simulink model "microgridbelbic"  (R2019a)
settings: Solver=VariableStepAuto  StartTime=0.0  StopTime=6  RelTol=1e-3
undefined symbols (not defined in the file): DiscIntNeverNeededParam, fdesignblkfcn, gcbh, Hydride, Metal, Nickel
libraries: powerlib x242, powerlib_extras x28, BELBICtoolbox x4, dsparch4 x1, electricdrivelib x1, simulink x1, sps_avr x1, powerlib_meascontrol x1, re_lib x1
(part 1 of 4)
settings Model: Creator=pavan  LastModifiedBy=pavan

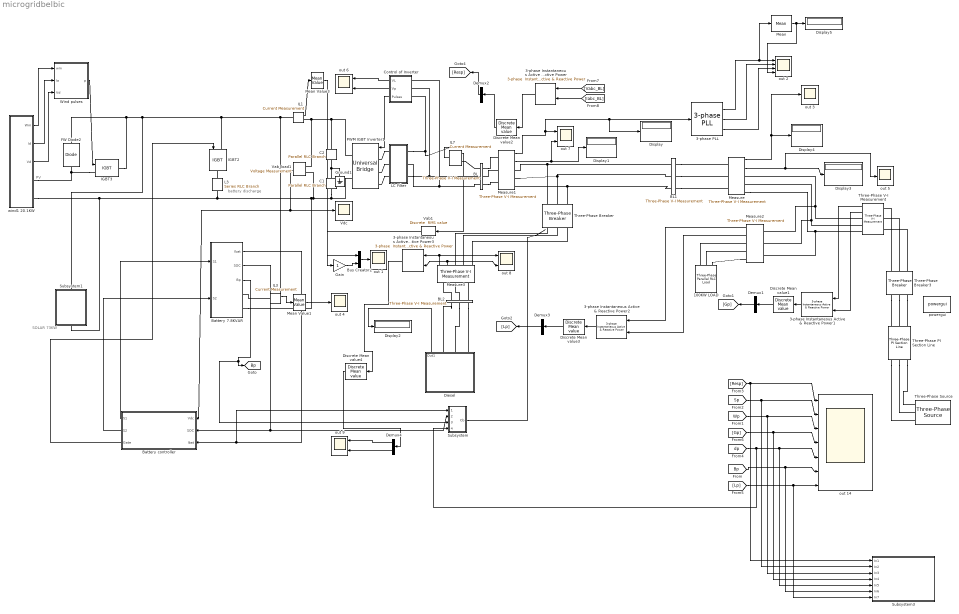
== system microgridbelbic ==
  note: SOLAR 73KW
  note: PV
  note: battery discharge
  100KW LOAD : powerlib/Elements/Three-Phase Parallel RLC Load  LConnTagsString=A|B|C  Configuration=Y (grounded)  NominalVoltage=400  Vabc=[1e3 1e3 1e3]  Vabcp=[1e3 1e3 1e3]  NominalFrequency=50  UnbalancedPower=off  ActivePower=80000  InductivePower=0  CapacitivePower=0  Pabc=[10e3 9e3 11e3]  QLabc=[100 90 110]  QCabc=[100 90 110]  Pabcp=[10e3 9e3 11e3]  QLabcp=[100 90 110]  QCabcp=[100 90 110]  Measurements=None  LoadType=constant Z
      settings: SourceProductName=Simscape Electrical
  3-phase Instantaneous Active & Reactive Power{,1..3} (4 alike) : powerlib_extras/Measurements/3-phase  Instantaneous  Active & Reactive Power
      settings: SourceProductName=Simscape Electrical  SourceProductBaseCode=PS
  3-phase PLL : powerlib_extras/Control  Blocks/3-phase PLL  Par_Init=[0 50]  ParK=[ 180 3200 1 ]  AGC=off
      settings: SourceProductName=Simscape Electrical  SourceProductBaseCode=PS
  BL : powerlib/Measurements/Three-Phase V-I Measurement  VoltageMeasurement=phase-to-ground  SetLabelV=on  LabelV=Vabc_BL1  Vpu=off  VpuLL=off  CurrentMeasurement=yes  SetLabelI=on  LabelI=Iabc_BL1  Ipu=off  Pbase=100e6  Vbase=500e3  OutputType=Magnitude  PhasorSimulation=off  PSBequivalent=0
      settings: SourceProductName=Simscape Electrical
  BL1 : powerlib/Measurements/Three-Phase V-I Measurement  VoltageMeasurement=phase-to-ground  SetLabelV=on  LabelV=Vabc_BL  Vpu=off  VpuLL=off  CurrentMeasurement=yes  SetLabelI=on  LabelI=Iabc_BL  Ipu=off  Pbase=100e6  Vbase=500e3  OutputType=Magnitude  PhasorSimulation=off  PSBequivalent=0
      settings: SourceProductName=Simscape Electrical
  BL2 : powerlib/Measurements/Three-Phase V-I Measurement  VoltageMeasurement=phase-to-ground  SetLabelV=on  LabelV=Vabc_BL2  Vpu=off  VpuLL=off  CurrentMeasurement=yes  SetLabelI=on  LabelI=Iabc_BL2  Ipu=off  Pbase=100e6  Vbase=500e3  OutputType=Magnitude  PhasorSimulation=off  PSBequivalent=0
      settings: SourceProductName=Simscape Electrical
  Battery controller : Subsystem
  "Battery 7.8KVAR " : Subsystem
  Bus Creator2 : BusCreator  Inputs=2
  C1 : powerlib/Elements/Parallel RLC Branch  LConnTagsString=a  RConnTagsString=__new0  BranchType=C  Resistance=1.0  Inductance=1.0  SetiL0=off  InitialCurrent=0  Capacitance=2200e-06*2  Setx0=off  InitialVoltage=0  Measurements=None
      settings: SourceProductName=Simscape Electrical
  C2 : powerlib/Elements/Parallel RLC Branch  LConnTagsString=a  RConnTagsString=__new0  BranchType=C  Resistance=1.0  Inductance=1.0  SetiL0=off  InitialCurrent=0  Capacitance=2200e-06*2  Setx0=off  InitialVoltage=0  Measurements=None
      settings: SourceProductName=Simscape Electrical
  Control of Inverter : Subsystem
  Demux1 : Demux  Outputs=1
  Demux2 : Demux  Outputs=1
  Demux3 : Demux  Outputs=1
  Demux4 : Demux  Outputs=2
  Diesel : Subsystem
  Discrete Mean value{1..4} (4 alike) : powerlib_extras/Discrete Measurements/Discrete  Mean value  Freq=50  Vinit=0  Ts=20e-6
      settings: SourceProductName=Simscape Electrical  SourceProductBaseCode=PS
  Display{,1..5} (6 alike) : Display
  FW Diode2 : powerlib/Power Electronics/Diode  Ron=0.01  Lon=0  Vf=0.8  IC=0  UseSnubber=off  Rs=100  Cs=0.1e-6  Measurements=off
      settings: SourceProductName=Simscape Electrical
  Gain : Gain
  Ground1 : powerlib/Elements/Ground  LConnTagsString=a
      settings: SourceProductName=Simscape Electrical
  IGBT2 : powerlib/Power Electronics/IGBT  Ron=0.001  Lon=0  Vf=1  Tf=1e-6  Tt=2e-6  IC=0  Rs=1e5  Cs=inf  Measurements=off
      settings: SourceProductName=Simscape Electrical
  IGBT3 : powerlib/Power Electronics/IGBT  Ron=0.001  Lon=0  Vf=1  Tf=1e-6  Tt=2e-6  IC=0  Rs=1e5  Cs=inf  Measurements=off
      settings: SourceProductName=Simscape Electrical
  IL1 : powerlib/Measurements/Current Measurement  PhasorSimulation=off  OutputType=Complex  PSBequivalent=0
      settings: SourceProductName=Simscape Electrical
  IL3 : powerlib/Measurements/Current Measurement  PhasorSimulation=off  OutputType=Complex  PSBequivalent=0
      settings: SourceProductName=Simscape Electrical
  IL7 : powerlib/Measurements/Current Measurement  PhasorSimulation=off  OutputType=Complex  PSBequivalent=0
      settings: SourceProductName=Simscape Electrical
  L3 : powerlib/Elements/Series RLC Branch  LConnTagsString=__new0  RConnTagsString=__new0  BranchType=R  Resistance=19  Inductance=2e-3  SetiL0=off  InitialCurrent=0  Capacitance=1.0  Setx0=off  InitialVoltage=0  Measurements=None
      settings: SourceProductName=Simscape Electrical
  LC Filter : Subsystem
  Mean : powerlib_meascontrol/Measurements/Mean  Freq=50  Vinit=0  Ts=0
      settings: SourceProductName=Simscape Electrical
  Mean Value1 : powerlib_extras/Measurements/Mean Value  Period=1/110
      settings: SourceProductName=Simscape Electrical  SourceProductBaseCode=PS
  Mean Value3 : powerlib_extras/Measurements/Mean Value  Period=1/110
      settings: SourceProductName=Simscape Electrical  SourceProductBaseCode=PS
  Measure : powerlib/Measurements/Three-Phase V-I Measurement  VoltageMeasurement=phase-to-ground  SetLabelV=off  LabelV=V1  Vpu=off  VpuLL=off  CurrentMeasurement=yes  SetLabelI=off  LabelI=I1  Ipu=off  Pbase=5.5e3  Vbase=385  OutputType=Magnitude  PhasorSimulation=off  PSBequivalent=0
      settings: SourceProductName=Simscape Electrical
  Measure1 : powerlib/Measurements/Three-Phase V-I Measurement  VoltageMeasurement=phase-to-ground  SetLabelV=off  LabelV=V1  Vpu=on  VpuLL=off  CurrentMeasurement=yes  SetLabelI=off  LabelI=I1  Ipu=on  Pbase=5.5e3  Vbase=385  OutputType=Magnitude  PhasorSimulation=off  PSBequivalent=0
      settings: SourceProductName=Simscape Electrical
  Measure2 : powerlib/Measurements/Three-Phase V-I Measurement  VoltageMeasurement=phase-to-ground  SetLabelV=off  LabelV=V1  Vpu=off  VpuLL=off  CurrentMeasurement=yes  SetLabelI=off  LabelI=I1  Ipu=off  Pbase=5.5e3  Vbase=385  OutputType=Magnitude  PhasorSimulation=off  PSBequivalent=0
      settings: SourceProductName=Simscape Electrical
  Measure3 : powerlib/Measurements/Three-Phase V-I Measurement  VoltageMeasurement=phase-to-ground  SetLabelV=off  LabelV=V1  Vpu=off  VpuLL=off  CurrentMeasurement=yes  SetLabelI=off  LabelI=I1  Ipu=off  Pbase=5.5e3  Vbase=385  OutputType=Magnitude  PhasorSimulation=off  PSBequivalent=0
      settings: SourceProductName=Simscape Electrical
  PWM IGBT Inverter1 : powerlib/Power Electronics/Universal Bridge  Arms=3  SnubberResistance=5000  SnubberCapacitance=inf  Device=IGBT / Diodes  Ron=1e-3  Lon=0  ForwardVoltages="[  0.0  0.0  ]"  ForwardVoltage=.8  GTOparameters=[ 1e-6 ,1e-6 ]  IGBTparameters=[ 1e-6 , 2e-6 ]  Measurements=Device currents  Measurements_2=None  converterType=Rectifier
      settings: SourceProductName=Simscape Electrical
  Subsystem : Subsystem
  Subsystem1 : Subsystem
  Subsystem3 : Subsystem
  Three-Phase PI Section Line : powerlib/Elements/Three-Phase PI Section Line  LConnTagsString=a|b|c  RConnTagsString=A|B|C  Frequency=50  Resistances=[ 0.01273 0.3864]  Inductances="[ 0.9337e-3  4.1264e-3]"  Capacitances=[12.74e-9 7.751e-9]  Length=100
      settings: SourceProductName=Simscape Electrical
  Three-Phase V-I Measurement : powerlib/Measurements/Three-Phase V-I Measurement  VoltageMeasurement=phase-to-ground  SetLabelV=off  LabelV=Vabc  Vpu=off  VpuLL=off  CurrentMeasurement=yes  SetLabelI=off  LabelI=Iabc  Ipu=off  Pbase=100e6  Vbase=500e3  OutputType=Complex  PhasorSimulation=off  PSBequivalent=0
      settings: SourceProductName=Simscape Electrical
  Three-Phase Breaker : powerlib/Elements/Three-Phase Breaker  InitialState=open  SwitchA=on  SwitchB=on  SwitchC=on  SwitchTimes=4  External=off  BreakerResistance=0.001  SnubberResistance=1e6  SnubberCapacitance=inf  Measurements=None
      settings: SourceProductName=Simscape Electrical
  Three-Phase Breaker3 : powerlib/Elements/Three-Phase Breaker  InitialState=closed  SwitchA=on  SwitchB=on  SwitchC=on  SwitchTimes=0  External=off  BreakerResistance=0.001  SnubberResistance=1e6  SnubberCapacitance=inf  Measurements=None
      settings: SourceProductName=Simscape Electrical
  Three-Phase Source : powerlib/Electrical Sources/Three-Phase Source  InternalConnection=Yg  VoltagePhases=off  Voltage=430  PhaseAngle=10  Voltage_phases=[25e3 25e3 25e3]/sqrt(3)  PhaseAngles_phases=[0 -120 +120]  Frequency=50  NonIdealSource=on  SpecifyImpedance=on  Resistance=0.8929  Inductance=16.58e-3  ShortCircuitLevel=100e6  BaseVoltage=25e3  XRratio=7  BusType=swing  Pref=10e3  Qref=0  Prefabc=[10e3, 10e3, 10e3]  Qrefabc=[0, 0, 0]  Qmin=-inf  Qmax=inf
      settings: SourceProductName=Simscape Electrical
  Vab1 : powerlib_extras/Discrete Measurements/Discrete  RMS value  Freq=50  Mag_Init=0  Ts=20e-6
      settings: SourceProductName=Simscape Electrical  SourceProductBaseCode=PS
  Vab_load1 : powerlib/Measurements/Voltage Measurement  Tag=PoWeRsYsTeMmEaSuReMeNt  PhasorSimulation=off  OutputType=Magnitude  PSBequivalent=0
      settings: SourceProductName=Simscape Electrical
  Vdc : Scope
  Wind pulses : Subsystem
  out {1,3..5} (4 alike) : Scope
  out 14 : Scope  NumInputPorts=7
  out 2 : Scope  NumInputPorts=4
  out {6..9} (4 alike) : Scope  NumInputPorts=2
  powergui : powerlib/powergui  Priority=1  SimulationMode=Discrete  SampleTime=10e-6  frequency=60  Iterations=50  frequencyindice=0  Pbase=100e6  ErrMax=1e-4  UnitsV=kV  UnitsW=MW  buscounter=0  FunctionMessages=off  echomessages=off  EnableUseOfTLC=off  CurrentSourceSwitches=off  DisableSnubberDevices=off  DisableRonSwitches=off  DisableVfSwitches=off  DisplayEquations=off  AutomaticDiscreteSolvers=off  SolverType=Tustin/Backward Euler (TBE)  Interpol=off  ExternalGateDelay=off  methode=off  Ts=0  x0status=blocks  SPID=off  SwTol=0  HookPort=off  NonlinearTolerance=0  nMaxIteration=15  ContinueOnMaxIteration=off  RestoreLinks=warning  ResistiveCurrentMeasurement=off  Frange=[0:2:500]  Ylog=off  Xlog=on  ShowGrid=off  save=off  variable=ZData  structure=Generator_Terminal  ZoomFFT=off  StartTime=0.0  cycles=1  DisplayStyle=1  fundamental=50  FreqAxis=off  MaxFrequency=4000  frequencyindicesteady=1  RmsSteady=1  display=off
      settings: SourceProductName=Simscape Electrical
  wind1 20.1KW : Subsystem
  tag scope: Bp=global
  wires:
  Discrete Mean value3/1 -> Demux3/1
  Diesel/1(Out1) -> Display2/1
  Control of Inverter/3(Pulses) -> PWM IGBT Inverter1/1
  Demux1/1 -> [Gp]
  Vab_load1/1 -> Battery controller/1(Vdc), Vdc/1
  [Vabc_BL] -> 3-phase Instantaneous Active & Reactive Power/1
  3-phase PLL/1 -> Mean/1, out 2/1
  Measure2/1 -> 3-phase Instantaneous Active & Reactive Power2/1
  [Lp] -> out 14/7, Subsystem3/7(In7)
  Discrete Mean value1/1 -> Demux1/1
  Measure3/2 -> 3-phase Instantaneous Active & Reactive Power3/2, out 8/2
  Mean Value1/1 -> out 4/1
  Demux3/1 -> [Lp]
  Demux4/1 -> out 9/1
  Measure/1 -> out 3/1, Display4/1
  Subsystem/1(Cb) -> ?
  Bus Creator2/1 -> out 1/1
  Measure3/1 -> 3-phase Instantaneous Active & Reactive Power3/1, out 8/1
  wind1 20.1KW/2(Id) -> Wind pulses/2(Ia)
  Vab1/1 -> Bus Creator2/1
  wind1 20.1KW/3(Vd) -> Wind pulses/3(Vd)
  Gain/1 -> Bus Creator2/2
  [Iabc_BL] -> 3-phase Instantaneous Active & Reactive Power/2
  IL7/1 -> Vab1/1
  Discrete Mean value4/1 -> Demux4/1
  Measure/2 -> out 5/1, Display3/1
  Control of Inverter/2(Vp) -> out 6/2
  Battery controller/1(S1) -> "Battery 7.8KVAR "/1(S1)
  Battery controller/3(Gate) -> IGBT2/1
  wind1 20.1KW/1(Wm) -> Wind pulses/1(wm)
  "Battery 7.8KVAR "/1(Ibat) -> Battery controller/3(Ibat), Subsystem/1(Ibat)
  Mean Value3/1 -> Gain/1
  IL1/1 -> Mean Value3/1
  3-phase Instantaneous Active & Reactive Power3/1 -> Discrete Mean value4/1
  Discrete Mean value2/1 -> Demux2/1
  3-phase Instantaneous Active & Reactive Power1/1 -> Discrete Mean value1/1
  Measure2/2 -> 3-phase Instantaneous Active & Reactive Power2/2
  Wind pulses/1(p) -> IGBT3/1
  "Battery 7.8KVAR "/3(Bp) -> [Bp], Subsystem/3(Vdc1)
  Three-Phase V-I Measurement/1 -> 3-phase Instantaneous Active & Reactive Power1/1
  [dp] -> Subsystem/4(Vdc2), out 14/5, Subsystem3/5(In5)
  [Sp] -> out 14/2, Subsystem3/2(In2)
  [Bp] -> out 14/6, Subsystem3/6(In6)
  Control of Inverter/1(VL) -> out 6/1
  Three-Phase V-I Measurement/2 -> 3-phase Instantaneous Active & Reactive Power1/2
  3-phase Instantaneous Active & Reactive Power/1 -> Discrete Mean value2/1
  [Resp] -> out 14/1, Subsystem3/1(In1)
  3-phase PLL/2 -> out 2/2
  Demux4/2 -> out 9/2
  [Wp] -> out 14/3, Subsystem3/3(In3)
  "Battery 7.8KVAR "/2(SOC) -> Battery controller/2(SOC), Subsystem/2(Soc)
  3-phase Instantaneous Active & Reactive Power2/1 -> Discrete Mean value3/1
  Battery controller/2(S2) -> "Battery 7.8KVAR "/2(S2)
  Measure1/1 -> out 7/1, Display/1, 3-phase PLL/1
  Measure1/2 -> Display1/1, out 7/2
  IL3/1 -> Mean Value1/1
  [Gp] -> out 14/4, Subsystem3/4(In4)
  Demux2/1 -> [Resp]
  3-phase PLL/3 -> out 2/3
  Mean/1 -> out 2/4, Display5/1
  connections:
  Measure/RConn3 -- Three-Phase V-I Measurement/RConn3 -- Measure2/LConn3
  Measure1/RConn2 -- Three-Phase Breaker/RConn2 -- BL1/LConn2
  BL1/LConn1 -- Three-Phase Breaker/RConn1 -- Measure1/RConn1
  IL1/RConn1 -- C2/LConn1 -- PWM IGBT Inverter1/RConn1 -- Vab_load1/LConn1
  Control of Inverter/LConn1 -- LC Filter/RConn3 -- BL/LConn3
  LC Filter/RConn1 -- IL7/LConn1 -- Control of Inverter/LConn3
  L3/RConn1 -- wind1 20.1KW/RConn2 -- Subsystem1/RConn1 -- "Battery 7.8KVAR "/RConn2 -- Vab_load1/LConn2 -- C1/RConn1 -- PWM IGBT Inverter1/RConn2
  Control of Inverter/LConn2 -- BL/LConn2 -- LC Filter/RConn2
  FW Diode2/RConn1 -- IL1/LConn1 -- IL3/RConn1 -- IGBT2/LConn1 -- Subsystem1/LConn1 -- IGBT3/RConn1
  Measure1/RConn3 -- Three-Phase Breaker/RConn3 -- BL1/LConn3
  C2/RConn1 -- C1/LConn1 -- Ground1/LConn1
  Three-Phase V-I Measurement/RConn1 -- Measure/RConn1 -- Measure2/LConn1
  IGBT3/LConn1 -- FW Diode2/LConn1 -- wind1 20.1KW/RConn1
  Three-Phase V-I Measurement/RConn2 -- Measure2/LConn2 -- Measure/RConn2
  Three-Phase Breaker3/LConn3 -- Three-Phase PI Section Line/LConn3
  BL1/RConn2 -- Measure/LConn2
  BL2/RConn2 -- Diesel/RConn2
  LC Filter/LConn3 -- PWM IGBT Inverter1/LConn3
  Three-Phase PI Section Line/RConn1 -- Three-Phase Source/RConn3
  BL/RConn3 -- Measure1/LConn3
  BL/RConn2 -- Measure1/LConn2
  Three-Phase Breaker3/LConn1 -- Three-Phase PI Section Line/LConn1
  BL2/LConn2 -- Measure3/LConn2
  Three-Phase Breaker3/RConn3 -- Three-Phase V-I Measurement/LConn3
  BL2/RConn1 -- Diesel/RConn1
  Measure2/RConn2 -- 100KW LOAD/LConn2
  LC Filter/LConn2 -- PWM IGBT Inverter1/LConn2
  Three-Phase PI Section Line/RConn3 -- Three-Phase Source/RConn1
  Three-Phase PI Section Line/RConn2 -- Three-Phase Source/RConn2
  Three-Phase Breaker3/LConn2 -- Three-Phase PI Section Line/LConn2
  Measure3/RConn3 -- Three-Phase Breaker/LConn3
  BL/RConn1 -- Measure1/LConn1
  IL3/LConn1 -- "Battery 7.8KVAR "/RConn1
  Measure3/RConn1 -- Three-Phase Breaker/LConn1
  BL/LConn1 -- IL7/RConn1
  Measure3/RConn2 -- Three-Phase Breaker/LConn2
  BL1/RConn3 -- Measure/LConn3
  Measure2/RConn1 -- 100KW LOAD/LConn1
  LC Filter/LConn1 -- PWM IGBT Inverter1/LConn1
  BL2/RConn3 -- Diesel/RConn3
  Three-Phase Breaker3/RConn1 -- Three-Phase V-I Measurement/LConn1
  Three-Phase Breaker3/RConn2 -- Three-Phase V-I Measurement/LConn2
  BL2/LConn1 -- Measure3/LConn1
  Measure2/RConn3 -- 100KW LOAD/LConn3
  BL1/RConn1 -- Measure/LConn1
  BL2/LConn3 -- Measure3/LConn3
  L3/LConn1 -- IGBT2/RConn1

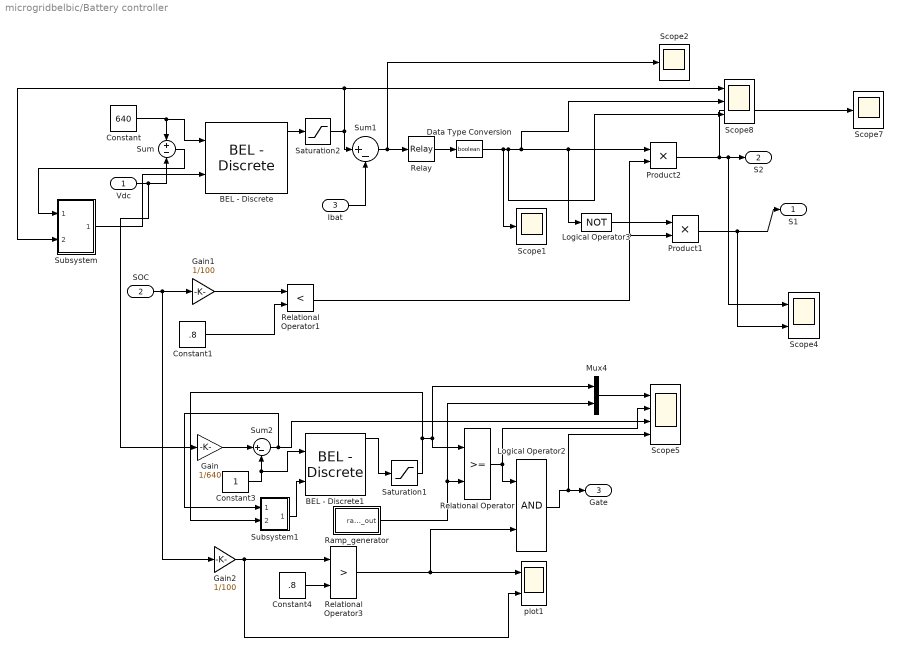
== system microgridbelbic/Battery controller ==
  Vdc : Inport
  SOC : Inport  Port=2
  Ibat : Inport  Port=3
  BEL - Discrete : BELBICtoolbox/Discrete-time/BEL - Discrete  alfa=0.5  beta=0.02  V=50  Vth=40  W=0.01  T=1
      settings: SourceProductName=BELBIC Toolbox
  BEL - Discrete1 : BELBICtoolbox/Discrete-time/BEL - Discrete  alfa=0.5  beta=0.001  V=50  Vth=10  W=0.01  T=1
      settings: SourceProductName=BELBIC Toolbox
  Constant : Constant  Value=640
  Constant1 : Constant  Value=.8
  Constant3 : Constant
  Constant4 : Constant  Value=.8
  Data Type Conversion : DataTypeConversion  OutDataTypeStr=boolean  RndMeth=Simplest  SaturateOnIntegerOverflow=on
  Gain : Gain  Gain=1/640  SaturateOnIntegerOverflow=on  OutDataTypeStr=Inherit: Same as input  ParamDataTypeStr=Inherit: Same as input
  Gain1 : Gain  Gain=1/100  SaturateOnIntegerOverflow=on  OutDataTypeStr=Inherit: Same as input  ParamDataTypeStr=Inherit: Same as input
  Gain2 : Gain  Gain=1/100  SaturateOnIntegerOverflow=on  OutDataTypeStr=Inherit: Same as input  ParamDataTypeStr=Inherit: Same as input
  Logical Operator2 : Logic
  Logical Operator3 : Logic  Operator=NOT
  Mux4 : Mux  Inputs=2
  Product1 : Product  RndMeth=Zero
  Product2 : Product  RndMeth=Zero
  Ramp_generator : Subsystem
  Relational Operator : RelationalOperator  RndMeth=Nearest  InputSameDT=on
  Relational Operator1 : RelationalOperator  Operator=<  RndMeth=Nearest  InputSameDT=on
  Relational Operator3 : RelationalOperator  Operator=>  RndMeth=Nearest  InputSameDT=on
  Relay : Relay  OnSwitchValue=2  OffSwitchValue=-2  OutDataTypeStr=Inherit: Inherit via back propagation
  Saturation1 : Saturate  UpperLimit=0.99  LowerLimit=0.1
  Saturation2 : Saturate  UpperLimit=0.99  LowerLimit=0.1
  Scope1 : Scope
  Scope2 : Scope
  Scope4 : Scope  NumInputPorts=2
  Scope5 : Scope  NumInputPorts=4
  Scope7 : Scope
  Scope8 : Scope  NumInputPorts=3
  Subsystem : Subsystem
  Subsystem1 : Subsystem
  Sum : Sum  Inputs=+-  SaturateOnIntegerOverflow=on  InputSameDT=on  OutDataTypeStr=Inherit: Same as first input
  Sum1 : Sum  Inputs=|+-  InputSameDT=on
  Sum2 : Sum  Inputs=|+-  SaturateOnIntegerOverflow=on  InputSameDT=on  OutDataTypeStr=Inherit: Same as first input
  plot1 : Scope  NumInputPorts=2
  S1 : Outport
  S2 : Outport  Port=2
  Gate : Outport  Port=3
  wires:
  BEL - Discrete/1 -> Saturation2/1
  Vdc/1 -> Sum/2, Gain/1
  Constant/1 -> BEL - Discrete/1, Sum/1
  Relay/1 -> Data Type Conversion/1
  Ibat/1 -> Sum1/2
  Sum1/1 -> Scope2/1, Relay/1
  Data Type Conversion/1 -> Scope8/2, Logical Operator3/1, Product2/1, Scope8/3, Scope1/1
  Gain1/1 -> Relational Operator1/1
  SOC/1 -> Gain1/1, Gain2/1
  Relational Operator1/1 -> Product2/2, Product1/2
  Constant1/1 -> Relational Operator1/2
  Product2/1 -> Scope7/1, S2/1, Scope4/1
  Relational Operator/1 -> Scope5/2, Logical Operator2/1
  Sum2/1 -> Scope5/3, Subsystem1/1(In1)
  Ramp_generator/1(ramp_out) -> Mux4/2, Relational Operator/2
  Mux4/1 -> Scope5/1
  BEL - Discrete1/1 -> Saturation1/1
  Relational Operator3/1 -> plot1/1, Logical Operator2/2
  Gain2/1 -> plot1/2, Relational Operator3/1
  Constant4/1 -> Relational Operator3/2
  Logical Operator2/1 -> Gate/1, Scope5/4
  Logical Operator3/1 -> Product1/1
  Product1/1 -> S1/1, Scope4/2
  Sum/1 -> Subsystem/1(In1)
  Subsystem/1(Out1) -> BEL - Discrete/2
  Constant3/1 -> BEL - Discrete1/1, Sum2/2
  Gain/1 -> Sum2/1
  Subsystem1/1(Out1) -> BEL - Discrete1/2
  Saturation1/1 -> Subsystem1/2(In2), Relational Operator/1, Mux4/1
  Saturation2/1 -> Subsystem/2(In2), Scope8/1, Sum1/1

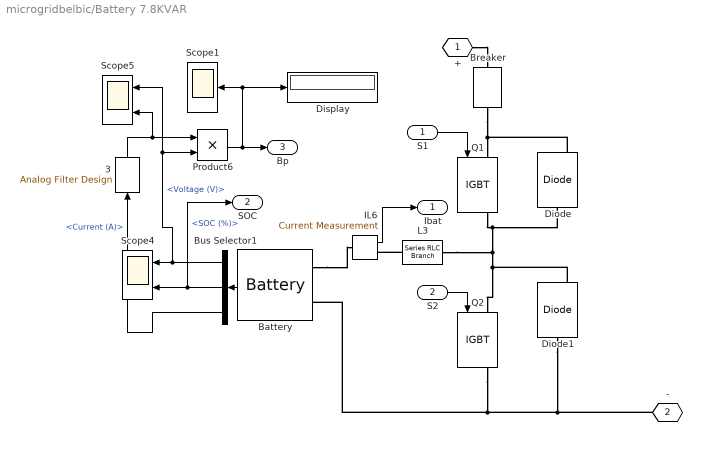
== system microgridbelbic/Battery 7.8KVAR  ==
  S1 : Inport
  S2 : Inport  Port=2
  3 : dsparch4/Analog Filter Design  method=Butterworth  filttype=Lowpass  N=8  Wlo=pi*50  Whi=80  Rp=2  Rs=40
  Battery : electricdrivelib/Extra Sources/Battery  BatType=Nickel-Metal-Hydride  ShowTempParam=off  ThermalPreset=no  ShowAgeParam=off  NomV=300  NomQ=6.5*4  SOC=60  Batt_Tr=30  PresetModel=on  MaxQ=28  MinV=225  FullV=353.3898  Dis_rate=5.2  R=0.11538  Normal_OP=25  expZone="[325.4237           5.2]"  current=[6.5 13 32.5]  Units=Time  Tci=20  NomT=20  T2=-30  MaxQ2=4.8  FullV2=7.1  Normal_OP2=5.655  expZone2="[6.58           1]"  Rca=0.6  ti=2000  Dp=0  Neq0=0  Tsim=1e6  Ta1=25  Qeol=5.4*0.9  Reol=0.013333*1.2  Char_age=[2.3478, 3]  Dis_age=[2.3478, 10]  N1=1500  N2=10500  N3=1000  N4=1400  Ta2=45  N5=950
      settings: SourceProductName=Simscape Electrical
  Breaker : powerlib/Elements/Breaker  InitialState=1  SwitchingTimes=[15 ]  External=off  BreakerResistance=0.01  SnubberResistance=1e6  SnubberCapacitance=inf  Measurements=None  MoreParameters=off  NoBreakLoop=off
      settings: SourceProductName=Simscape Electrical
  Bus Selector1 : BusSelector  OutputSignals=Voltage (V),SOC (%),Current (A)
  Diode : powerlib/Power Electronics/Diode  Ron=0.001  Lon=0  Vf=0.8  IC=0  UseSnubber=off  Rs=500  Cs=250e-9  Measurements=on
      settings: SourceProductName=Simscape Electrical
  Diode1 : powerlib/Power Electronics/Diode  Ron=0.001  Lon=0  Vf=0.8  IC=0  UseSnubber=off  Rs=500  Cs=250e-9  Measurements=on
      settings: SourceProductName=Simscape Electrical
  Display : Display
  IL6 : powerlib/Measurements/Current Measurement  PhasorSimulation=off  OutputType=Complex  PSBequivalent=0
      settings: SourceProductName=Simscape Electrical
  L3 : powerlib/Elements/Series RLC Branch  LConnTagsString=__new0  RConnTagsString=__new0  BranchType=L  Resistance=1.0  Inductance=5e-3  SetiL0=off  InitialCurrent=0  Capacitance=1.0  Setx0=off  InitialVoltage=0  Measurements=None
      settings: SourceProductName=Simscape Electrical
  Product6 : Product  RndMeth=Zero
  Q1 : powerlib/Power Electronics/IGBT  Ron=0.001  Lon=0  Vf=1  Tf=1e-6  Tt=2e-6  IC=0  Rs=1e5  Cs=inf  Measurements=on
      settings: SourceProductName=Simscape Electrical
  Q2 : powerlib/Power Electronics/IGBT  Ron=0.001  Lon=0  Vf=1  Tf=1e-6  Tt=2e-6  IC=0  Rs=1e5  Cs=inf  Measurements=on
      settings: SourceProductName=Simscape Electrical
  Scope1 : Scope
  Scope4 : Scope  NumInputPorts=2
  Scope5 : Scope  NumInputPorts=2
  + : PMIOPort  Tag=PMCPort  Side=Right
  - : PMIOPort  Tag=PMCPort  Port=2  Side=Right
  Ibat : Outport
  SOC : Outport  Port=2
  Bp : Outport  Port=3
  wires:
  Bus Selector1/1 -> Scope4/1, Product6/2, Scope5/1  "<Voltage (V)>"
  Bus Selector1/2 -> Scope4/2, SOC/1  "<SOC (%)>"
  Bus Selector1/3 -> 3/1  "<Current (A)>"
  Product6/1 -> Bp/1, Display/1, Scope1/1
  S1/1 -> Q1/1
  S2/1 -> Q2/1
  IL6/1 -> Ibat/1
  3/1 -> Product6/1, Scope5/2
  Battery/1 -> Bus Selector1/1
  connections:
  Battery/LConn2 -- Q2/RConn1 -- -/RConn1 -- Diode1/LConn1
  +/RConn1 -- Breaker/LConn1
  Breaker/RConn1 -- Diode/RConn1 -- Q1/LConn1
  Q2/LConn1 -- Diode1/RConn1 -- L3/RConn1 -- Diode/LConn1 -- Q1/RConn1
  L3/LConn1 -- IL6/RConn1
  Battery/LConn1 -- IL6/LConn1

== system microgridbelbic/Control of Inverter ==
  note: Control of Inverter
  Discrete PWM Generator1 : Subsystem  AncestorBlock=|  DialogController=POWERSYS.PowerSysDialog  mask(Discrete PWM Generator){GeneratorMode=3-arm  bridge (6 pulses), Fc=4000, Ts=20e-6, Internal=off, mIndex=0.4, Freq=60, Phase=0}
      | powerlib_extras/Discrete 
      | Control Blocks/Discrete
      | PWM Generator
      mask prompts: GeneratorMode "Generator Mode"; Fc "Carrier frequency (Hz):"; Ts "Sample time:"; Internal "Internal generation of modulating signal(s)"; mIndex "Modulation index  (0<m<1) :"; Freq "Frequency of output voltage (Hz)"; Phase "Phase of output voltage (degrees)"
      mask help:
      | This discrete block generates pulses for carrier-based PWM (Pulse Width Modulation), self-commutated IGBTs,GTOs or FETs bridges.
      |
      | Depending on the number of bridge arms selected in the "Generator Mode" parameter, the block can be used either for single-phase or three-phase PWM control.
      mask init:
      | powericon('psbcallbacks',gcb,'Discrete PWM Generator');
      | if Freq==0
      |     Phase=90;
      | end
      | switch GeneratorMode
      | case 1,
      |     Internal_Phase=0;
      |    Signal_PortWidth=1;
      |    Select1_Elements=[1 2];
      |    Select1_PortWidth=2;
      |    Select3_Elements=[1 2];
      |    Select3_PortWidth=4;
      | case 2,
      |     Internal_Phase=0;
      |     Signal_PortWidth=1;
      |     Select1_Elements=[1 2];
      |     Select1_PortWidth=2;
      |     Select3_Elements=[1 2 3 4];
      |     Select3_PortWidth=4;
      | case 3,
      |     Internal_Phase=[0 -2*pi/3 2*pi/3];
      |     Signal_PortWidth=3;
      |     Select1_Elements=[1 4 2 5 3 6];
      |     Select1_PortWidth=6;
      |    Select3_Elements=[1 2 3 4 5 6];
      |    Select3_PortWidth=12;
      | case 4,
      |     Internal_Phase=[0 -2*pi/3 2*pi/3];
      |     Signal_PortWidth=3;
      |     Select1_Elements=[1 4 2 5 3 6];
      |     Select1_PortWidth=6;
      |    Select3_Elements=[1 2 3 4 5 6 7 8 9 10 11 12];
      |    Select3_PortWidth=12;
      | end
      | power_initmask();
      mask Help:
      | The output pulses are a vector (with values=0 or 1). Depending on the selected "Generator Mode", the output vector contains:
      | For a 1-arm  bridge: Two pulses. Pulse 1 is for the upper switch and pulse 2 is for the lower switch.
      | For a 2-arm  bridge: Four pulses. Pulses 1 and 3 are respectively for the upper switches of the first and second arm. Pulses 2 and 4 are for the lower switches.
      | For a 3-arm  bridge: Six pulses. Pulses 1,3 and 5 are respectively for the upper switches of the first,second and third arm. Pulses 2,4 and 6 are for the lower switches.
      | For double 3-arm bridges: Twelve pulses.The first six pulses (pulses 1 to 6) must be sent to the first 3-arm bridge and the last six (pulses 7 to 12) to the second 3-arm bridge.
      | 
      | By selecting "Internal generation" you can can control the modulation index m, frequency and phase of the output voltage  from the internal parameters (m, Freq and Phase). Otherwise, external signals are used for pulse generation. The width of the input vector must be 1 for single phase bridges ( 1-arm or 2-arm)  and 3 for 3-phase bridges  (single or double bridge).
      mask TypeOptions GeneratorMode: 1-arm  bridge (2 pulses) | 2-arm  bridge (4 pulses) | 3-arm  bridge (6 pulses) | Double 3-arm  bridges (12 pulses)
      mask Callback Internal: powericon('psbcallbacks',gcb,'Discrete PWM Generator',[]);
  MI Controller : Subsystem
  Subsystem1 : Subsystem
  Unit Delay4 : UnitDelay  SampleTime=20e-6
  VL-L : Scope
  Vph_rms : Scope
  Vph_rms1 : Scope
  C : PMIOPort  Side=Left
  B : PMIOPort  Port=2  Side=Left
  A : PMIOPort  Port=3  Side=Left
  VL : Outport
  Vp : Outport  Port=2
  Pulses : Outport  Port=3
  wires:
  Unit Delay4/1 -> Pulses/1
  Discrete PWM Generator1/1(Pulses) -> Unit Delay4/1
  MI Controller/1(Vabc_inv) -> Vph_rms1/1, Discrete PWM Generator1/1(Uref)
  Subsystem1/1(Vph) -> MI Controller/1(Vabc)
  Subsystem1/2(VL-L) -> VL-L/1, VL/1
  Subsystem1/3(Vph_rms) -> Vph_rms/1, Vp/1
  connections:
  A/RConn1 -- Subsystem1/LConn1
  B/RConn1 -- Subsystem1/LConn2
  C/RConn1 -- Subsystem1/LConn3

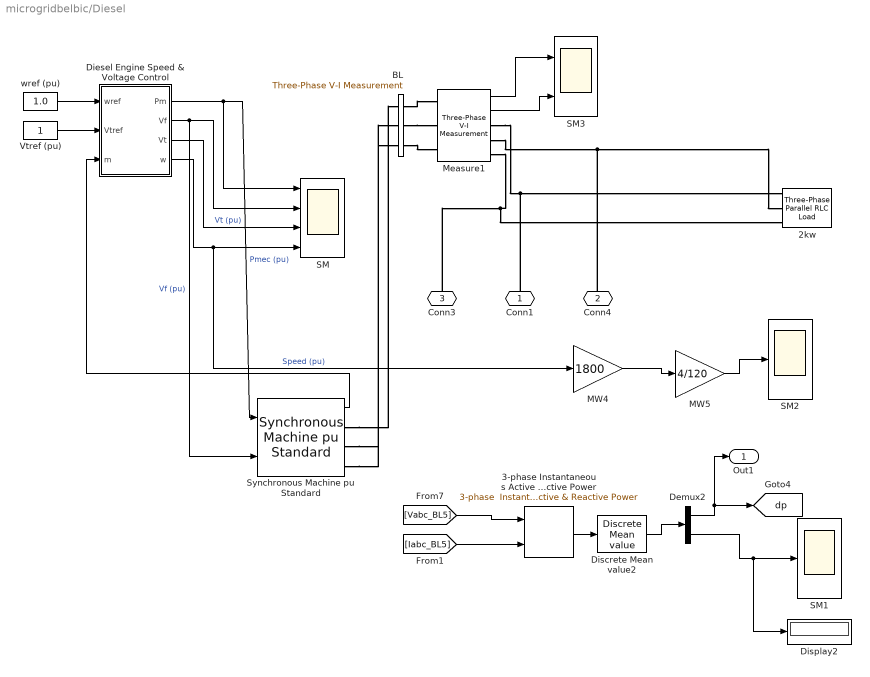
== system microgridbelbic/Diesel ==
  2kw : powerlib/Elements/Three-Phase Parallel RLC Load  LConnTagsString=A|B|C  Configuration=Y (grounded)  NominalVoltage=600  Vabc=[1e3 1e3 1e3]  Vabcp=[1e3 1e3 1e3]  NominalFrequency=50  UnbalancedPower=off  ActivePower=500  InductivePower=0  CapacitivePower=0  Pabc=[10e3 9e3 11e3]  QLabc=[100 90 110]  QCabc=[100 90 110]  Pabcp=[10e3 9e3 11e3]  QLabcp=[100 90 110]  QCabcp=[100 90 110]  Measurements=None  LoadType=constant Z
      settings: SourceProductName=Simscape Electrical
  3-phase Instantaneous Active & Reactive Power : powerlib_extras/Measurements/3-phase  Instantaneous  Active & Reactive Power
      settings: SourceProductName=Simscape Electrical  SourceProductBaseCode=PS
  BL : powerlib/Measurements/Three-Phase V-I Measurement  VoltageMeasurement=phase-to-ground  SetLabelV=on  LabelV=Vabc_BL5  Vpu=off  VpuLL=off  CurrentMeasurement=yes  SetLabelI=on  LabelI=Iabc_BL5  Ipu=off  Pbase=100e6  Vbase=500e3  OutputType=Magnitude  PhasorSimulation=off  PSBequivalent=0
      settings: SourceProductName=Simscape Electrical
  Demux2 : Demux  Outputs=2
  Diesel Engine Speed & Voltage Control : Subsystem
  Discrete Mean value2 : powerlib_extras/Discrete Measurements/Discrete  Mean value  Freq=50  Vinit=0  Ts=20e-6
      settings: SourceProductName=Simscape Electrical  SourceProductBaseCode=PS
  Display2 : Display
  MW4 : Gain  Gain=1800  SaturateOnIntegerOverflow=on  OutDataTypeStr=Inherit: Same as input  ParamDataTypeStr=Inherit: Same as input
  MW5 : Gain  Gain=4/120  SaturateOnIntegerOverflow=on  OutDataTypeStr=Inherit: Same as input  ParamDataTypeStr=Inherit: Same as input
  Measure1 : powerlib/Measurements/Three-Phase V-I Measurement  VoltageMeasurement=phase-to-ground  SetLabelV=off  LabelV=V1  Vpu=off  VpuLL=off  CurrentMeasurement=yes  SetLabelI=off  LabelI=I1  Ipu=off  Pbase=5.5e3  Vbase=385  OutputType=Magnitude  PhasorSimulation=off  PSBequivalent=0
      settings: SourceProductName=Simscape Electrical
  SM : Scope  NumInputPorts=4
  SM1 : Scope
  SM2 : Scope
  SM3 : Scope  NumInputPorts=2
  Synchronous Machine pu Standard : powerlib/Machines/Synchronous Machine pu Standard  PresetModel=01: 50Hz 400V 8.1kVA 1500RPM  MechanicalLoad=Mechanical power Pm  ShowDetailedParameters=on  RotorType=Salient-pole  Units=per unit standard parameters  MeasurementBus=off  NominalParameters=[8100 400 50]  Reactances1=[ 1.81, 0.3, 0.23, 1.76, 0.65, 0.25, 0.15 ]  Reactances2=[1.8 0.184 0.115 0.895 0.207 0.072]  dAxisTimeConstants=Short-circuit  qAxisTimeConstants=Short-circuit  TimeConstants1="[ 4.4849  0.0681  0.1  ]"  TimeConstants2=[ 8.0, 0.03, 1.0, 0.07 ]  TimeConstants3="[  3.7  0.05  0.05  ]"  TimeConstants4=[ 8.0, 0.03, 0.3371, 0.0295 ]  TimeConstants5=[ 1.01, 0.053, 0.1 ]  TimeConstants6=[ 1.3201, 0.023, 1.0, 0.07 ]  TimeConstants7=[0.012 0.003 0.003]  TimeConstants8=[ 1.3201, 0.0231, 0.3371, 0.0295 ]  StatorResistance=0.0820125  Mechanical=[0.1406 0.02742 2]  PolePairs=2  InitialConditions="[ 0  0  0  0  0  0  0  0  1 ]"  SetSaturation=off  Saturation=[0.6404,0.7127,0.8441,0.9214,0.9956,1.082,1.19,1.316,1.457;0.7,0.7698,0.8872,0.9466,0.9969,1.046,1.1,1.151,1.201]  LoadFlowParameters=[1,0,0,0,0]  TsPowergui=0  TsBlock=-1  IterativeModel=Forward Euler  IterativeDiscreteModel=Trapezoidal non iterative  BusType=PV  Pref=0  Qref=0  Qmin=-inf  Qmax=inf  PLF=0  QLF=0
      settings: SourceProductName=Simscape Electrical
  Vtref (pu) : Constant
  wref (pu) : Constant  Value=1.0
  Conn1 : PMIOPort  Side=Right
  Conn4 : PMIOPort  Port=2  Side=Right
  Conn3 : PMIOPort  Port=3  Side=Right
  Out1 : Outport
  tag scope: dp=global
  wires:
  wref (pu)/1 -> Diesel Engine Speed & Voltage Control/1(wref)
  Vtref (pu)/1 -> Diesel Engine Speed & Voltage Control/2(Vtref)
  Diesel Engine Speed & Voltage Control/3(Vt) -> SM/3  "Vt (pu)"
  Diesel Engine Speed & Voltage Control/4(w) -> SM/4, MW4/1  "Speed (pu)"
  Diesel Engine Speed & Voltage Control/1(Pm) -> SM/1, Synchronous Machine pu Standard/1  "Pmec (pu)"
  Diesel Engine Speed & Voltage Control/2(Vf) -> SM/2, Synchronous Machine pu Standard/2  "Vf (pu)"
  3-phase Instantaneous Active & Reactive Power/1 -> Discrete Mean value2/1
  MW4/1 -> MW5/1
  MW5/1 -> SM2/1
  Discrete Mean value2/1 -> Demux2/1
  Demux2/1 -> [dp], Out1/1
  Demux2/2 -> SM1/1, Display2/1
  [Vabc_BL5] -> 3-phase Instantaneous Active & Reactive Power/1
  [Iabc_BL5] -> 3-phase Instantaneous Active & Reactive Power/2
  Measure1/1 -> SM3/1
  Measure1/2 -> SM3/2
  Synchronous Machine pu Standard/1 -> Diesel Engine Speed & Voltage Control/3(m)
  connections:
  Measure1/RConn1 -- 2kw/LConn1 -- Conn1/RConn1
  Measure1/RConn2 -- 2kw/LConn2 -- Conn4/RConn1
  Measure1/RConn3 -- 2kw/LConn3 -- Conn3/RConn1
  BL/RConn1 -- Measure1/LConn1
  BL/RConn2 -- Measure1/LConn2
  BL/RConn3 -- Measure1/LConn3
  Synchronous Machine pu Standard/RConn1 -- BL/LConn1
  Synchronous Machine pu Standard/RConn2 -- BL/LConn2
  Synchronous Machine pu Standard/RConn3 -- BL/LConn3

== system microgridbelbic/LC Filter ==
  "2 mH " : powerlib/Elements/Three-Phase Series RLC Branch  LConnTagsString=A|B|C  RConnTagsString=A|B|C  BranchType=L  Resistance=1.0  Inductance=2.7193e-4  Capacitance=1.0  Measurements=None
      settings: SourceProductName=Simscape Electrical
  Ground : powerlib/Elements/Ground  LConnTagsString=a
      settings: SourceProductName=Simscape Electrical
  Ground1 : powerlib/Elements/Ground  LConnTagsString=a
      settings: SourceProductName=Simscape Electrical
  Ground2 : powerlib/Elements/Ground  LConnTagsString=a
      settings: SourceProductName=Simscape Electrical
  Three-Phase Series RLC Branch : powerlib/Elements/Three-Phase Series RLC Branch  LConnTagsString=A|B|C  RConnTagsString=A|B|C  BranchType=C  Resistance=.1  Inductance=1e-3  Capacitance=8.7186e-5  Measurements=None
      settings: SourceProductName=Simscape Electrical
  A : PMIOPort  Side=Left
  B : PMIOPort  Port=2  Side=Left
  C : PMIOPort  Port=3  Side=Left
  "A " : PMIOPort  Port=4  Side=Right
  "B " : PMIOPort  Port=5  Side=Right
  "C " : PMIOPort  Port=6  Side=Right
  connections:
  B/RConn1 -- "2 mH "/LConn2
  A/RConn1 -- "2 mH "/LConn1
  C/RConn1 -- "2 mH "/LConn3
  "2 mH "/RConn1 -- "A "/RConn1 -- Three-Phase Series RLC Branch/LConn1
  "2 mH "/RConn2 -- "B "/RConn1 -- Three-Phase Series RLC Branch/LConn2
  "2 mH "/RConn3 -- "C "/RConn1 -- Three-Phase Series RLC Branch/LConn3
  Ground/LConn1 -- Three-Phase Series RLC Branch/RConn1
  Ground1/LConn1 -- Three-Phase Series RLC Branch/RConn2
  Ground2/LConn1 -- Three-Phase Series RLC Branch/RConn3

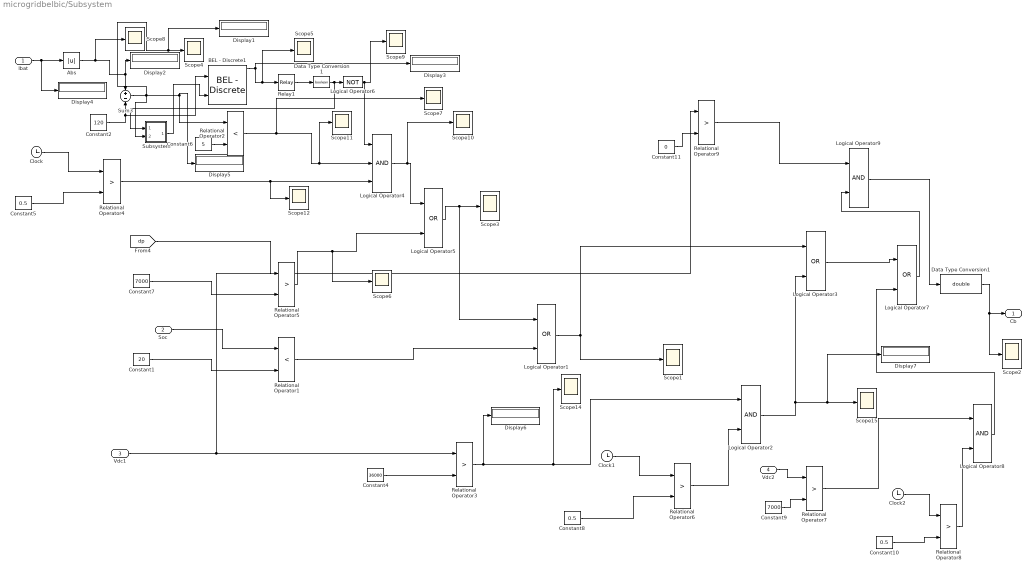
== system microgridbelbic/Subsystem ==
  Ibat : Inport
  Soc : Inport  Port=2
  Vdc1 : Inport  Port=3
  Vdc2 : Inport  Port=4
  Abs : Abs
  BEL - Discrete1 : BELBICtoolbox/Discrete-time/BEL - Discrete  alfa=0.1  beta=0.05  V=300  Vth=200  W=0.1  T=1
      settings: SourceProductName=BELBIC Toolbox
  Clock : Clock
  Clock1 : Clock
  Clock2 : Clock
  Constant1 : Constant  Value=20
  Constant10 : Constant  Value=0.5
  Constant11 : Constant  Value=0
  Constant2 : Constant  Value=120
  Constant4 : Constant  Value=36000
  Constant5 : Constant  Value=0.5
  Constant6 : Constant  Value=5
  Constant7 : Constant  Value=7000
  Constant8 : Constant  Value=0.5
  Constant9 : Constant  Value=7000
  Data Type Conversion1 : DataTypeConversion  OutDataTypeStr=boolean  RndMeth=Simplest  SaturateOnIntegerOverflow=on
  Data Type Conversion1 : DataTypeConversion  OutDataTypeStr=double
  Display{1..7} (7 alike) : Display
  Logical Operator{1,3,5,7} (4 alike) : Logic  Operator=OR
  Logical Operator2 : Logic
  Logical Operator4 : Logic  Inputs=3
  Logical Operator6 : Logic  Operator=NOT
  Logical Operator8 : Logic
  Logical Operator9 : Logic
  Relational Operator1 : RelationalOperator  Operator=<  RndMeth=Nearest  InputSameDT=on
  Relational Operator2 : RelationalOperator  Operator=<  RndMeth=Nearest  InputSameDT=on
  Relational Operator{3..9} (7 alike) : RelationalOperator  Operator=>  RndMeth=Nearest  InputSameDT=on
  Relay1 : Relay  OnSwitchValue=10  OffSwitchValue=-10  OutDataTypeStr=Inherit: Inherit via back propagation
  Scope{1..12,14..15} (14 alike) : Scope
  Subsystem : Subsystem
  Sum3 : Sum  Inputs=+-  SaturateOnIntegerOverflow=on  InputSameDT=on  OutDataTypeStr=Inherit: Same as first input
  Cb : Outport
  wires:
  Constant2/1 -> Sum3/2, BEL - Discrete1/1
  Sum3/1 -> Display5/1, Relational Operator2/1, Scope4/1, Display1/1, Subsystem/2(In2)
  Constant6/1 -> Relational Operator2/2
  BEL - Discrete1/1 -> Relay1/1, Scope5/1, Display3/1
  Clock/1 -> Relational Operator4/1
  Constant5/1 -> Relational Operator4/2
  Relational Operator2/1 -> Logical Operator4/2, Scope11/1, Scope7/1
  Relational Operator4/1 -> Logical Operator4/3, Scope12/1
  [dp] -> Relational Operator5/1
  Constant7/1 -> Relational Operator5/2
  Relational Operator5/1 -> Logical Operator5/2, Scope6/1
  Logical Operator4/1 -> Logical Operator5/1, Scope10/1
  Logical Operator5/1 -> Logical Operator1/1, Scope3/1
  Data Type Conversion1/1 -> Subsystem/1(In1), Logical Operator6/1
  Logical Operator6/1 -> Scope9/1, Logical Operator4/1
  Soc/1 -> Relational Operator1/1
  Constant1/1 -> Relational Operator1/2
  Relational Operator1/1 -> Logical Operator1/2
  Logical Operator1/1 -> Scope1/1, Logical Operator3/1
  Ibat/1 -> Display4/1, Abs/1
  Constant4/1 -> Relational Operator3/2
  Clock1/1 -> Relational Operator6/1
  Constant8/1 -> Relational Operator6/2
  Relational Operator3/1 -> Logical Operator2/1, Scope14/1, Display6/1
  Relational Operator6/1 -> Logical Operator2/2
  Logical Operator2/1 -> Scope15/1, Display7/1, Logical Operator3/2
  Vdc1/1 -> Relational Operator3/1, Relational Operator9/1
  Vdc2/1 -> Relational Operator7/1
  Constant9/1 -> Relational Operator7/2
  Logical Operator3/1 -> Logical Operator7/1
  Data Type Conversion1/1 -> Cb/1, Scope2/1
  Clock2/1 -> Relational Operator8/1
  Constant10/1 -> Relational Operator8/2
  Relational Operator7/1 -> Logical Operator8/1
  Relational Operator8/1 -> Logical Operator8/2
  Logical Operator8/1 -> Logical Operator7/2
  Constant11/1 -> Relational Operator9/2
  Relational Operator9/1 -> Logical Operator9/1
  Logical Operator7/1 -> Logical Operator9/2
  Logical Operator9/1 -> Data Type Conversion1/1
  Abs/1 -> Scope8/1, Sum3/1, Display2/1
  Subsystem/1(Out1) -> BEL - Discrete1/2
  Relay1/1 -> Data Type Conversion1/1

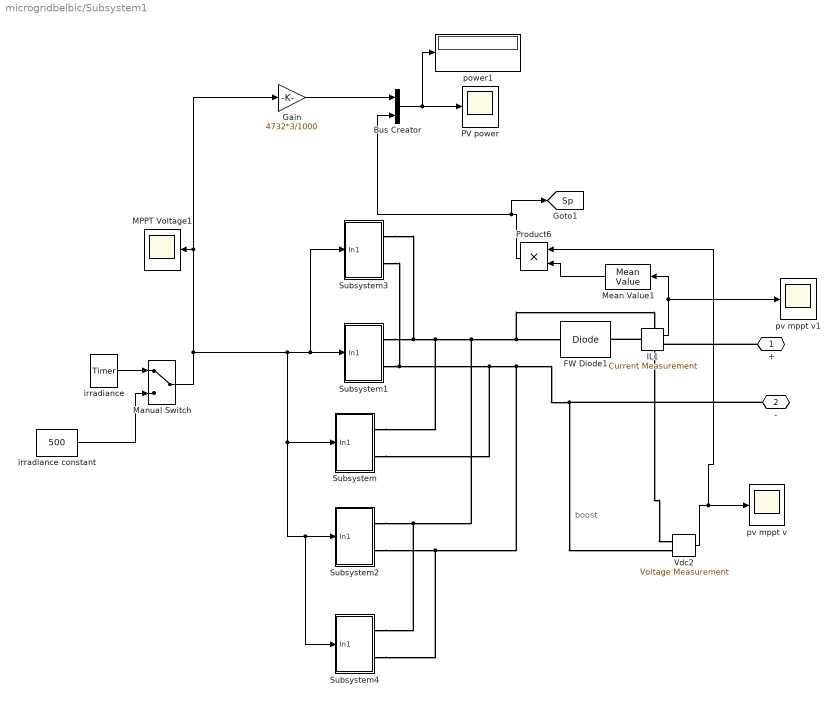
== system microgridbelbic/Subsystem1 ==
  note: boost
  Bus Creator : BusCreator  Inputs=2
  FW Diode1 : powerlib/Power Electronics/Diode  Ron=0.01  Lon=0  Vf=0.8  IC=0  UseSnubber=off  Rs=100  Cs=0.1e-6  Measurements=off
      settings: SourceProductName=Simscape Electrical
  Gain : Gain  Gain=4732*3/1000
  IL1 : powerlib/Measurements/Current Measurement  PhasorSimulation=off  OutputType=Complex  PSBequivalent=0
      settings: SourceProductName=Simscape Electrical
  MPPT Voltage1 : Scope
  Manual Switch : ManualSwitch
  Mean Value1 : powerlib_extras/Measurements/Mean Value  Period=0.0045
      settings: SourceProductName=Simscape Electrical  SourceProductBaseCode=PS
  PV power : Scope
  Product6 : Product  RndMeth=Zero
  Subsystem : Subsystem
  Subsystem1 : Subsystem
  Subsystem2 : Subsystem
  Subsystem3 : Subsystem
  Subsystem4 : Subsystem
  Vdc2 : powerlib/Measurements/Voltage Measurement  Tag=PoWeRsYsTeMmEaSuReMeNt  PhasorSimulation=off  OutputType=Magnitude  PSBequivalent=0
      settings: SourceProductName=Simscape Electrical
  irradiance : powerlib_extras/Control  Blocks/Timer  t=[0 2 4 ]  e=[1000 850 700]
      settings: SourceProductName=Simscape Electrical  SourceProductBaseCode=PS
  irradiance constant : Constant  Value=500  SampleTime=20e-6
  power1 : Display
      settings: SampleTime=1e-3
  pv mppt v : Scope
  pv mppt v1 : Scope
  + : PMIOPort  Side=Left
  - : PMIOPort  Port=2  Side=Right
  tag scope: Sp=global
  wires:
  IL1/1 -> pv mppt v1/1, Mean Value1/1
  Mean Value1/1 -> Product6/2
  irradiance constant/1 -> Manual Switch/2
  irradiance/1 -> Manual Switch/1
  Bus Creator/1 -> power1/1, PV power/1
  Gain/1 -> Bus Creator/1
  Product6/1 -> [Sp], Bus Creator/2
  Manual Switch/1 -> Gain/1, MPPT Voltage1/1, Subsystem3/1(In1), Subsystem1/1(In1), Subsystem4/1(In1), Subsystem2/1(In1), Subsystem/1(In1)
  Vdc2/1 -> Product6/1, pv mppt v/1
  connections:
  Subsystem1/RConn2 -- Subsystem/RConn2 -- -/RConn1 -- Vdc2/LConn2 -- Subsystem4/RConn2 -- Subsystem2/RConn2 -- Subsystem3/RConn2
  +/RConn1 -- IL1/RConn1
  IL1/LConn1 -- FW Diode1/RConn1
  Subsystem4/RConn1 -- Subsystem3/RConn1 -- Subsystem1/RConn1 -- Subsystem/RConn1 -- Vdc2/LConn1 -- FW Diode1/LConn1 -- Subsystem2/RConn1

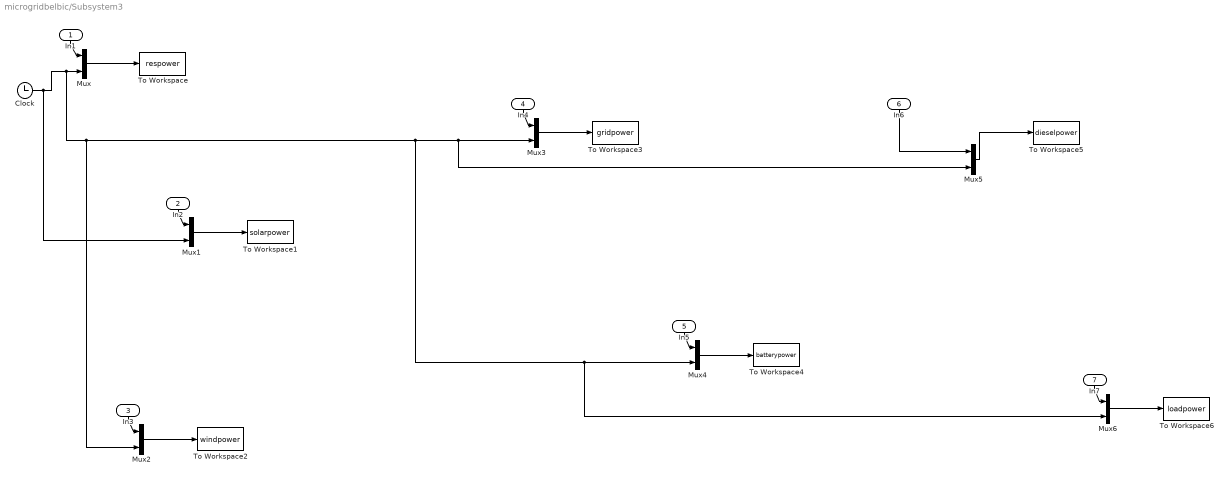
== system microgridbelbic/Subsystem3 ==
  In1 : Inport
  In2 : Inport  Port=2
  In3 : Inport  Port=3
  In4 : Inport  Port=4
  In5 : Inport  Port=5
  In6 : Inport  Port=6
  In7 : Inport  Port=7
  Clock : Clock
  Mux{,1..6} (7 alike) : Mux  Inputs=2
  To Workspace : ToWorkspace  VariableName=respower  SampleTime=-1
  To Workspace1 : ToWorkspace  VariableName=solarpower  SampleTime=-1
  To Workspace2 : ToWorkspace  VariableName=windpower  SampleTime=-1
  To Workspace3 : ToWorkspace  VariableName=gridpower  SampleTime=-1
  To Workspace4 : ToWorkspace  VariableName=batterypower  SampleTime=-1
  To Workspace5 : ToWorkspace  VariableName=dieselpower  SampleTime=-1
  To Workspace6 : ToWorkspace  VariableName=loadpower  SampleTime=-1
  wires:
  Mux/1 -> To Workspace/1
  Clock/1 -> Mux1/2, Mux/2, Mux3/2, Mux5/2, Mux4/2, Mux6/2, Mux2/2
  In1/1 -> Mux/1
  Mux1/1 -> To Workspace1/1
  In2/1 -> Mux1/1
  Mux2/1 -> To Workspace2/1
  In3/1 -> Mux2/1
  Mux3/1 -> To Workspace3/1
  In4/1 -> Mux3/1
  Mux4/1 -> To Workspace4/1
  In5/1 -> Mux4/1
  Mux5/1 -> To Workspace5/1
  In6/1 -> Mux5/1
  Mux6/1 -> To Workspace6/1
  In7/1 -> Mux6/1

== system microgridbelbic/Wind pulses ==
  wm : Inport
  Ia : Inport  Port=2
  Vd : Inport  Port=3
  Current Controller1 : Subsystem  mask{h=0.1}
      mask prompts: h "Hysteresis band (A)"
      mask help: Hysteresis Current Controller
      mask Display: plot(0,0,100,100,[45,45],[35,65],[55,55],[35,65],[45,65],[65,65],[35,55],[35,35])
  Discrete 1st-Order Filter2 : powerlib_extras/Discrete  Control Blocks/Discrete 1st-Order Filter  FilterType=Lowpass  Tc=100e-3  Ts=20e-6  Initialize=off  Vac_Init=[0.8 -25 60]  Vdc_Init=-0.4  PlotResponse=off  param1=[1 500 0.1]
      settings: SourceProductName=Simscape Electrical  SourceProductBaseCode=PS
  Subsystem : Subsystem
  Torque reference 1 : Subsystem
  Unit Delay3 : UnitDelay  SampleTime=-1
  genertaor terminal1 : Scope  NumInputPorts=2
  p : Outport
  wires:
  Current Controller1/2(error1) -> genertaor terminal1/2
  Ia/1 -> Unit Delay3/1
  Vd/1 -> Subsystem/3(Vd)
  wm/1 -> Subsystem/2(wm), Torque reference 1/1(wm)
  Current Controller1/1(g) -> genertaor terminal1/1, p/1
  Discrete 1st-Order Filter2/1 -> Current Controller1/1(Iref)
  Subsystem/1(Id_ref) -> Discrete 1st-Order Filter2/1
  Torque reference 1/1(Tref) -> Subsystem/1(Tref)
  Unit Delay3/1 -> Current Controller1/2(Ia)

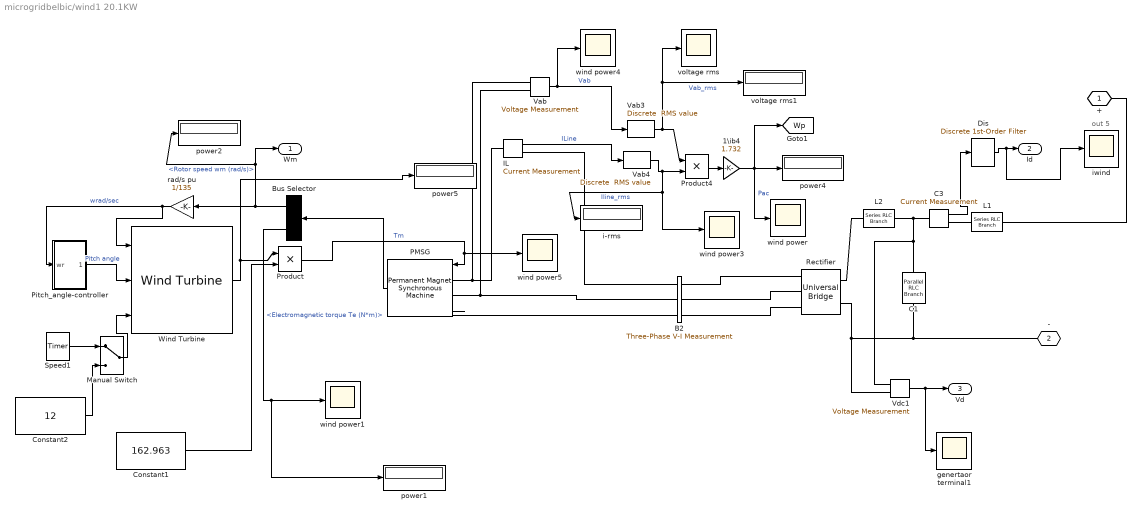
== system microgridbelbic/wind1 20.1KW ==
  note: out 5
  1\ib4 : Gain  Gain=1.732  SaturateOnIntegerOverflow=on  OutDataTypeStr=Inherit: Same as input  ParamDataTypeStr=Inherit: Same as input
  "B2 " : powerlib/Measurements/Three-Phase V-I Measurement  VoltageMeasurement=no  SetLabelV=on  LabelV=Vabc_B2  Vpu=off  VpuLL=off  CurrentMeasurement=no  SetLabelI=on  LabelI=Iabc_B2  Ipu=off  Pbase=100e6  Vbase=500e3  OutputType=Magnitude  PhasorSimulation=off  PSBequivalent=0
      settings: SourceProductName=Simscape Electrical
  Bus Selector : BusSelector  OutputSignals=Rotor speed wm (rad/s),Electromagnetic torque Te (N*m)
  C1 : powerlib/Elements/Parallel RLC Branch  LConnTagsString=a  RConnTagsString=__new0  BranchType=C  Resistance=1.0  Inductance=1.0  SetiL0=off  InitialCurrent=0  Capacitance=1000e-06  Setx0=off  InitialVoltage=650  Measurements=None
      settings: SourceProductName=Simscape Electrical
  C3 : powerlib/Measurements/Current Measurement  PhasorSimulation=off  OutputType=Complex  PSBequivalent=0
      settings: SourceProductName=Simscape Electrical
  Constant1 : Constant  Value=162.963
  Constant2 : Constant  Value=12
  Dis : powerlib_extras/Discrete  Control Blocks/Discrete 1st-Order Filter  FilterType=Lowpass  Tc=100e-3  Ts=20e-6  Initialize=off  Vac_Init=[0.8 -25 60]  Vdc_Init=-0.4  PlotResponse=off  param1=[1 500 0.1]
      settings: SourceProductName=Simscape Electrical  SourceProductBaseCode=PS
  IL : powerlib/Measurements/Current Measurement  PhasorSimulation=off  OutputType=Complex  PSBequivalent=0
      settings: SourceProductName=Simscape Electrical
  L1 : powerlib/Elements/Series RLC Branch  LConnTagsString=__new0  RConnTagsString=__new0  BranchType=L  Resistance=1.0  Inductance=2e-3  SetiL0=off  InitialCurrent=0  Capacitance=1.0  Setx0=off  InitialVoltage=0  Measurements=None
      settings: SourceProductName=Simscape Electrical
  L2 : powerlib/Elements/Series RLC Branch  LConnTagsString=__new0  RConnTagsString=__new0  BranchType=L  Resistance=1.0  Inductance=2e-3  SetiL0=off  InitialCurrent=0  Capacitance=1.0  Setx0=off  InitialVoltage=0  Measurements=None
      settings: SourceProductName=Simscape Electrical
  Manual Switch : ManualSwitch
  PMSG : powerlib/Machines/Permanent Magnet Synchronous Machine  NbPhases=3  FluxDistribution=Sinusoidal  RotorType=Round  MechanicalLoad=Torque Tm  PresetModel=No  ShowDetailedParameters=on  MeasurementBus=off  Resistance=0.425  Inductance=8.5e-3  dqInductances=[0.0082 0.0082]  La=0.000395  MachineConstant=Flux linkage established by magnets (V.s)  Flux=0.55  VoltageCst=698.3128  TorqueCst=5.775  Flat=120  Mechanical=[0.01197 0.001189 7]  PolePairs=7  InitialConditions=[0,0, 0,0]  InitialConditions5ph=[0 0 0 0 0 0]  TsPowergui=0  TsBlock=-1  RefAngle=90 degrees behind phase A axis (modified Park)
  Pitch_angle-controller : Subsystem
  Product : Product  RndMeth=Zero
  Product4 : Product  RndMeth=Zero
  Rectifier : powerlib/Power Electronics/Universal Bridge  Arms=3  SnubberResistance=100  SnubberCapacitance=0.1e-6  Device=Diodes  Ron=1e-3  Lon=0  ForwardVoltages="[  0.8  0.8  ]"  ForwardVoltage=.8  GTOparameters=[ 10e-6 , 20e-6 ]  IGBTparameters=[ 1e-6 , 2e-6 ]  Measurements=Device currents  Measurements_2=None  converterType=Rectifier
      settings: SourceProductName=Simscape Electrical
  Speed1 : powerlib_extras/Control  Blocks/Timer  t=[0 2 6 ]  e=[9 13 12]
      settings: SourceProductName=Simscape Electrical  SourceProductBaseCode=PS
  Vab : powerlib/Measurements/Voltage Measurement  PhasorSimulation=off  OutputType=Complex  PSBequivalent=0
      settings: SourceProductName=Simscape Electrical
  Vab3 : powerlib_extras/Discrete Measurements/Discrete  RMS value  Freq=50  Mag_Init=0  Ts=20e-6
      settings: SourceProductName=Simscape Electrical  SourceProductBaseCode=PS
  Vab4 : powerlib_extras/Discrete Measurements/Discrete  RMS value  Freq=50  Mag_Init=0  Ts=20e-6
      settings: SourceProductName=Simscape Electrical  SourceProductBaseCode=PS
  Vdc1 : powerlib/Measurements/Voltage Measurement  Tag=PoWeRsYsTeMmEaSuReMeNt  PhasorSimulation=off  OutputType=Magnitude  PSBequivalent=0
      settings: SourceProductName=Simscape Electrical
  Wind Turbine : re_lib/Wind Generation/Wind Turbine  Pnom=20000  Pelec_base=120000/0.9  wind_base=12  P_wind_base=0.8  speed_nom=1  pitch_angle=0  c1_c6="[0.51763          116          0.4            5           21     0.006795]"  cp_nom=0.48  lambda_nom=8.1
      settings: SourceProductName=Simscape Electrical  SourceProductBaseCode=PS
  genertaor terminal1 : Scope
  i-rms : Display
      settings: SampleTime=1e-3
  iwind : Scope
  power{1..2,4..5} (4 alike) : Display
      settings: SampleTime=1e-3
  rad/s pu : Gain  Gain=1/135  SaturateOnIntegerOverflow=on  OutDataTypeStr=Inherit: Same as input  ParamDataTypeStr=Inherit: Same as input
  voltage rms : Scope
  voltage rms1 : Display
      settings: SampleTime=1e-3
  wind power{,1,3..5} (5 alike) : Scope
  + : PMIOPort  Tag=PMCPort  Side=Right
  - : PMIOPort  Tag=PMCPort  Port=2  Side=Right
  Wm : Outport
  Id : Outport  Port=2
  Vd : Outport  Port=3
  tag scope: Wp=global
  wires:
  Dis/1 -> iwind/1, Id/1
  C3/1 -> Dis/1
  PMSG/1 -> Bus Selector/1
  Pitch_angle-controller/1(Pitch_angle) -> Wind Turbine/2  "Pitch angle"
  Vdc1/1 -> Vd/1, genertaor terminal1/1
  1\ib4/1 -> [Wp], wind power/1, power4/1  "Pac"
  Vab4/1 -> i-rms/1, wind power3/1, Product4/2  "Iline_rms"
  Vab3/1 -> voltage rms1/1, voltage rms/1, Product4/1  "Vab_rms"
  Product/1 -> wind power5/1, PMSG/1  "Tm"
  Product4/1 -> 1\ib4/1
  IL/1 -> Vab4/1  "ILine"
  Vab/1 -> Vab3/1, wind power4/1  "Vab"
  rad/s pu/1 -> Wind Turbine/1, Pitch_angle-controller/1(wr)  "wrad/sec"
  Bus Selector/1 -> rad/s pu/1, power2/1, Wm/1  "<Rotor speed wm (rad/s)>"
  Constant1/1 -> Product/2
  Wind Turbine/1 -> power5/1, Product/1
  Bus Selector/2 -> wind power1/1, power1/1  "<Electromagnetic torque Te (N*m)>"
  Speed1/1 -> Manual Switch/1
  Constant2/1 -> Manual Switch/2
  Manual Switch/1 -> Wind Turbine/3
  connections:
  L1/RConn1 -- +/RConn1
  L2/LConn1 -- Rectifier/RConn1
  PMSG/LConn1 -- IL/LConn1 -- Vab/LConn1
  C3/RConn1 -- L1/LConn1
  L2/RConn1 -- C1/LConn1 -- Vdc1/LConn1 -- C3/LConn1
  Rectifier/RConn2 -- Vdc1/LConn2 -- C1/RConn1 -- -/RConn1
  "B2 "/RConn3 -- Rectifier/LConn3
  Rectifier/LConn2 -- "B2 "/RConn2
  "B2 "/RConn1 -- Rectifier/LConn1
  PMSG/LConn3 -- "B2 "/LConn3
  Vab/LConn2 -- PMSG/LConn2 -- "B2 "/LConn2
  "B2 "/LConn1 -- IL/RConn1

== system microgridbelbic/Battery controller/Ramp_generator ==
  note: Carrier Freq
  Constant3 : Constant
  Discrete-Time Integrator1 : DiscreteIntegrator  ExternalReset=rising  SampleTime=20e-6  ICPrevOutput=DiscIntNeverNeededParam  ICPrevScaledInput=DiscIntNeverNeededParam
  Relational Operator1 : RelationalOperator  RndMeth=Nearest  InputSameDT=on
  Unit Delay1 : UnitDelay  SampleTime=20e-6
  fc : Constant  Value=10000
  ramp_out : Outport
  wires:
  Unit Delay1/1 -> Discrete-Time Integrator1/2
  Relational Operator1/1 -> Unit Delay1/1
  Constant3/1 -> Relational Operator1/2
  Discrete-Time Integrator1/1 -> ramp_out/1, Relational Operator1/1
  fc/1 -> Discrete-Time Integrator1/1

== system microgridbelbic/Battery controller/Subsystem ==
  In1 : Inport
  In2 : Inport  Port=2
  Add : Sum
  Gain1 : Gain  Gain=0.2
  Gain2 : Gain  Gain=0.04
  Out1 : Outport
  wires:
  In1/1 -> Gain1/1
  Gain2/1 -> Add/2
  In2/1 -> Gain2/1
  Add/1 -> Out1/1
  Gain1/1 -> Add/1

== system microgridbelbic/Battery controller/Subsystem1 ==
  In1 : Inport
  In2 : Inport  Port=2
  Add : Sum
  Gain1 : Gain  Gain=0.2
  Gain2 : Gain  Gain=0.01
  Out1 : Outport
  wires:
  In1/1 -> Gain1/1
  Gain2/1 -> Add/2
  In2/1 -> Gain2/1
  Add/1 -> Out1/1
  Gain1/1 -> Add/1
